simulink model "Funcion"  (R2020a)
settings: Solver=FixedStepAuto  StartTime=0.0  StopTime=10.0  RelTol=1e-3
libraries: androiduilib x4
settings Model: Creator=luisi  LastModifiedBy=luisi
settings OptimizationCC: EnhancedBackFolding=on  PassReuseOutputArgsAs=Individual arguments  ZeroExternalMemoryAtStartup=off  ZeroInternalMemoryAtStartup=off  MaxStackSize=64  OptimizeBlockOrder=speed  DifferentSizesBufferReuse=on  OptimizationCustomize=off  EfficientTunableParamExpr=on
settings DebuggingCC: ParameterTunabilityLossMsg=error
settings HardwareCC: ProdBitPerPointer=32  ProdBitPerSizeT=32  ProdBitPerPtrDiffT=32  ProdLargestAtomicInteger=Long  ProdLargestAtomicFloat=Double  ProdWordSize=32  ProdHWDeviceType=ARM Compatible->ARM Cortex
settings SFSimCC: MATLABDynamicMemAlloc=off
settings RTWCC: SystemTargetFile=ert.tlc  HardwareBoard=Android Device  TemplateMakefile=ert_default_tmf  RTWVerbose=off  Toolchain=Android SDK/NDK Tools
settings CodeAppCC: ForceParamTrailComments=on  IgnoreCustomStorageClasses=off  OperatorAnnotations=on  SimulinkDataObjDesc=on  SFDataObjDesc=on  InsertBlockDesc=on

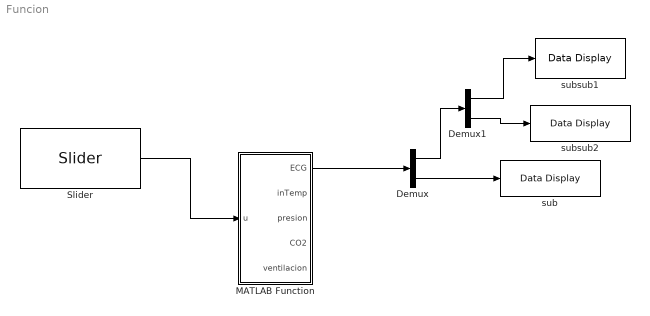
== system Funcion ==
  Demux : Demux  Outputs=2
  Demux1 : Demux  Outputs=2
  MATLAB Function : MATLAB Function  TreatAsAtomicUnit=on
  Slider : androiduilib/Slider  Min=0  Value=0  Max=2  Resolution=1  SliderId=Funcion/Slider  SampleTime=0.1  BlockPlatform=Android
      settings: SourceProductBaseCode=ANDROID
  sub : androiduilib/Data Display  DataDisplayId=Funcion/sub  Format=Float  Precision=6  SimulateUsing=Code generation  blockPlatform=Android
      settings: SourceProductBaseCode=ANDROID
  subsub1 : androiduilib/Data Display  DataDisplayId=Funcion/subsub1  Format=Float  Precision=6  SimulateUsing=Code generation  blockPlatform=Android
      settings: SourceProductBaseCode=ANDROID
  subsub2 : androiduilib/Data Display  DataDisplayId=Funcion/subsub2  Format=Float  Precision=6  SimulateUsing=Code generation  blockPlatform=Android
      settings: SourceProductBaseCode=ANDROID
  wires:
  Slider/1 -> MATLAB Function/1(u)
  MATLAB Function/1(ECG) -> Demux/1
  Demux/1 -> Demux1/1
  Demux/2 -> sub/1
  Demux1/2 -> subsub2/1
  Demux1/1 -> subsub1/1

== matlab function Funcion/MATLAB Function ==
  data: ECG output; u input; inTemp output; presion output; CO2 output; ventilacion output
function  [ECG, inTemp, presion, CO2, ventilacion]= fcn(u)
if u==1
   %% ECG (no segmento ST y R peq)
     %ECG = [alphaP, alphaQ, picoR, alphaS, alphaT, thetaT, omegaECG, GananciaOut, offsetMaxFinder]
    alphaP= 0.6; %Valor de magnitud pico onda P
    alphaQ=-5;  %Valor de magnitud pico onda Q
    picoR=10;  %Valor de magnitud pico onda R
    alphaS=-7.5; %Valor de magnitud pico onda S
    alphaT=0.75*0.5; %Valor de magnitud pico onda T
    thetaT = pi/3; % Angulo donde se ubica la onda T
    omegaECG=8; %Frecuencia angular ECG
    gananciaOut= 0.7;   
    
    %%% TEMP (fiebre)
    inTemp= 1;%1.05;
    
    %%Presion
    Re0=0.0160;
    Ra=0.06; Rlv=1.2; Rv=0.016; Rem=10; 
    Ce=1.5;Ca=1.5;Cv=50;
    c1=0.1; c2=6; c3=0.01;c4=500; c5=18.4207; c6=7.5;
    Ed=0.06;Es0=3;
    epsilon=0.00001;
    A1=0.5; 
    omega0=7.54;
        
    %% CO2 (baja saturacion)
    phi=15; %valor max de saturacion
    tau1=0.2; %tiempo subida inspiracion
    tau2=0.1; %tiempo subida espiracion
    d=2;  %Periodo
    alphaCo2=1;  % Factor de relacion de magnitudes
    
    %% Ventilacion (mayor frec)
    Ci=0.1;
    Ri= 16.41;
    tf = 2; %duración total del ciclo    
    ti=1;  %tiempo de inspiración
    Vt= 0.5;  %% valor maximo de onda de respiracion. Volumen aire en litros
    
elseif u==0
    
    %% ECG    
    alphaP= 0.6; %Valor de magnitud pico onda P
    alphaQ=-5;  %Valor de magnitud pico onda Q
    picoR=18;  %Valor de magnitud pico onda R
    alphaS=-7.5; %Valor de magnitud pico onda S
    alphaT=0.75*0.5; %Valor de magnitud pico onda T
    thetaT = 4*pi/6; % Angulo donde se ubica la onda T
    omegaECG=8; %Frecuencia angular ECG
    gananciaOut= 0.7;  %Valor para escalar salida del modelo    
    
    %%% TEMP
    inTemp= 0;%1;
    
    %%Presion
    Re0=0.0055222;Ra=0.025; Rlv=0.41279; Rv=0.02;
    Ce=1.69;Ca=2;Cv=15;
    c1=0.01; c2=4.0153; c3=0.000498;c4=150; c5=18.445;c6=1;
    Ed=0.0655; Es0=0.57; Rem=10.009; epsilon=0.00001; A1=0.40341; 
    omega0=8.37;
        
    %% CO2
    phi=32; %valor max de saturacion
    tau1=0.2; %tiempo subida inspiracion
    tau2=0.1; %tiempo subida espiracion
    d=2;  %Periodo
    alphaCo2=1;  % Factor de relacion de magnitudes
    
    %% Ventilacion
    Ci=0.1;
    Ri=16.41;
    tf = 4; %duración total del ciclo
    ti=2;  %tiempo de inspiración
    Vt= 1.03;
       
else
    
    %% ECG    
    alphaP= 0.6; %Valor de magnitud pico onda P
    alphaQ=-5;  %Valor de magnitud pico onda Q
    picoR=18;  %Valor de magnitud pico onda R
    alphaS=-7.5; %Valor de magnitud pico onda S
    alphaT=0.75*0.5; %Valor de magnitud pico onda T
    thetaT = pi/3; % Angulo donde se ubica la onda T
    omegaECG=8; %Frecuencia angular ECG
    gananciaOut= 0.7;  %Valor para escalar salida del modelo    
    
    %%% TEMP
    inTemp= 3%0.95;
    
    %%Presion
    Re0=0.0055222;Ra=0.025; Rlv=0.41279; Rv=0.02;
    Ce=1.69;Ca=2;Cv=15;
    c1=0.01; c2=4.0153; c3=0.000498;c4=150; c5=18.445;c6=1;
    Ed=0.0655; Es0=0.57; Rem=10.009; epsilon=0.00001; A1=0.40341; 
    omega0=8.37;
        
    %% CO2
    phi=32; %valor max de saturacion
    tau1=0.2; %tiempo subida inspiracion
    tau2=0.1; %tiempo subida espiracion
    d=2;  %Periodo
    alphaCo2=1;  % Factor de relacion de magnitudes
    
    %% Ventilacion
    Ci=0.1;
    Ri=16.41;
    tf = 4; %duración total del ciclo
    ti=2;  %tiempo de inspiración
    Vt= 1.03;
    
    
end
offsetMaxFinder= (picoR)*gananciaOut*0.0045/0.7;
Tsys= 0.3333*2*pi/omega0;
Tdia= (1-0.3333)*2*pi/omega0;
Tpresion =Tsys+Tdia;
A = exp(ti/(Ri*Ci));
B= exp(tf/(Ri*Ci));
Pex= -(Vt*A)/(Ci*(A-B));
D= exp(-ti/(Ri*Ci));
Pset= Pex+(Vt/(D*(A-1)*Ci));
    
ECG=[alphaP,alphaQ, picoR, alphaS, alphaT, thetaT, omegaECG,gananciaOut, offsetMaxFinder ];
presion=[Re0, Ra, Rlv, Rv, c1, c2, c3, c4, c5, c6,Ed, Ce, Ca, Cv, Es0, Rem, epsilon, A1, omega0, Tsys, Tdia, Tpresion];
CO2=[phi,tau1,tau2,d,alphaCo2];
ventilacion =[Ci, Ri, tf, Pex, Pset]; %falta condicion inicial y tiempos ti tf
